simulink model "multip_1"  (Simulink 7.8)
settings: Solver=ode45  StartTime=0.0  StopTime=10.0  RelTol=1e-3
values from neighbouring files (symbols this model uses):
  Vb = 117.5643    [addition_1.m]    (also in addition_11.m; addition_2.m; addition_21.m; addition_3.m)
  Vc = -69.1715    [addition_1.m]    (also in addition_11.m; addition_2.m; addition_21.m; addition_3.m)
settings Model: Creator=svenhoffmann  LastModifiedBy=josef  ExtModeAutoUpdateStatusClock=off
settings DataIOCC: SignalLoggingName=sigsOut
settings OptimizationCC: InlineInvariantSignals=on  InitFltsAndDblsToZero=on
settings DebuggingCC: SaveWithParameterizedLinksMsg=none  SignalResolutionControl=TryResolveAllWithWarning  SolverPrmCheckMsg=none  MultiTaskDSMMsg=warning  MultiTaskCondExecSysMsg=none  FcnCallInpInsideContextMsg=Use local settings  StrictBusMsg=None
settings HardwareCC: TargetUnknown=on
settings RTWCC: IncludeERTFirstTime=on
settings GRTTargetCC: TargetFcnLib=ansi_tfl_tmw.mat

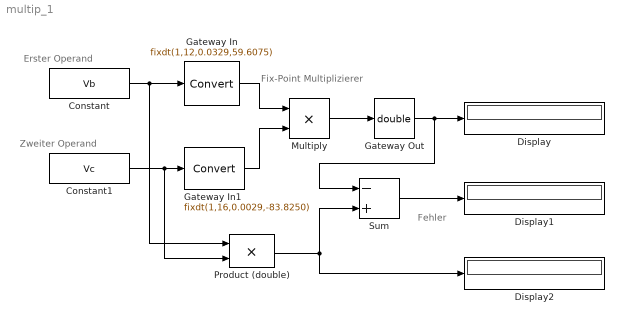
== system multip_1 ==
  note: Erster Operand
  note: Zweiter Operand
  note: Fix-Point
      | Multiplizierer
  note: Fehler
  Constant : Constant  Value=Vb
  Constant1 : Constant  Value=Vc
  Display : Display
  Display1 : Display
  Display2 : Display
  Gateway In : DataTypeConversion  OutDataTypeStr=fixdt(1,12,0.0329,59.6075)  RndMeth=Nearest  SaturateOnIntegerOverflow=on
  Gateway In1 : DataTypeConversion  OutDataTypeStr=fixdt(1,16,0.0029,-83.8250)  RndMeth=Nearest
  Gateway Out : DataTypeConversion  OutDataTypeStr=double
  Multiply : Product  Inputs=**  OutDataTypeStr=slDataTypeAndScale(('sfix(nba)'),('[Sa, Ba]'))  RndMeth=Nearest
  Product (double) : Product  SaturateOnIntegerOverflow=on  OutDataTypeStr=Inherit: Same as first input
  Sum : Sum  Inputs=-+  SaturateOnIntegerOverflow=on
  wires:
  Constant/1 -> Gateway In/1, Product (double)/1
  Constant1/1 -> Product (double)/2, Gateway In1/1
  Gateway In/1 -> Multiply/1
  Gateway In1/1 -> Multiply/2
  Multiply/1 -> Gateway Out/1
  Gateway Out/1 -> Display/1, Sum/1
  Product (double)/1 -> Sum/2, Display2/1
  Sum/1 -> Display1/1
